simulink model "simuMF"  (R2021a)
settings: Solver=VariableStepAuto  StartTime=0.0  StopTime=100000  RelTol=1e-3
values from neighbouring files (symbols this model uses):
  C1 = tf(C1)    [control.m]
  C2 = tf(C2)    [control.m]
  H = tf(0.0001867, [1 0.0001919])    [control.m]
  pi_cd = tf(pi)    [control.m]
  pif = tf([39.15 0.06366], [1 0])    [control.m]
libraries: simulink x1
settings Model: Creator=jricl  LastModifiedBy=jricl

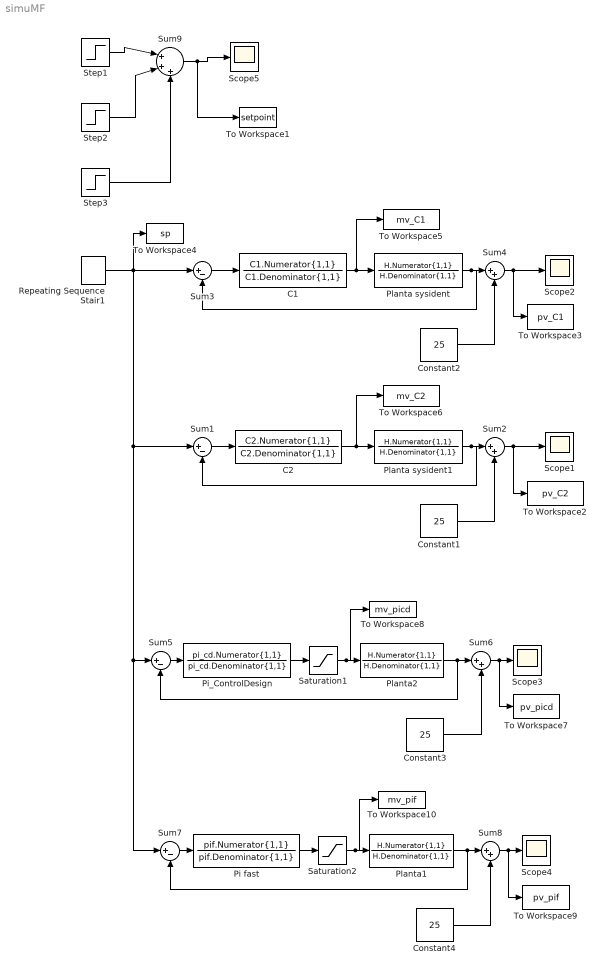
== system simuMF ==
  C1 : TransferFcn  Numerator=C1.Numerator{1,1}  Denominator=C1.Denominator{1,1}
  C2 : TransferFcn  Numerator=C2.Numerator{1,1}  Denominator=C2.Denominator{1,1}
  Constant{1..4} (4 alike) : Constant  Value=25
  Pi fast : TransferFcn  Numerator=pif.Numerator{1,1}  Denominator=pif.Denominator{1,1}
  Pi_ControlDesign : TransferFcn  Numerator=pi_cd.Numerator{1,1}  Denominator=pi_cd.Denominator{1,1}
  Planta sysident : TransferFcn  Numerator=H.Numerator{1,1}  Denominator=H.Denominator{1,1}
  Planta sysident1 : TransferFcn  Numerator=H.Numerator{1,1}  Denominator=H.Denominator{1,1}
  Planta1 : TransferFcn  Numerator=H.Numerator{1,1}  Denominator=H.Denominator{1,1}
  Planta2 : TransferFcn  Numerator=H.Numerator{1,1}  Denominator=H.Denominator{1,1}
  Repeating Sequence Stair1 : simulink/Sources/Repeating Sequence Stair  OutValues=[5 10 15 20]  tsamp=25000  OutMin=[]  OutMax=[]  OutDataTypeStr=double  OutputDataTypeScalingMode=double  OutDataType=fixdt(0,8)  ConRadixGroup=Best Precision: Vector-wise  OutScaling=2^-12
  Saturation1 : Saturate  UpperLimit=100  LowerLimit=0
  Saturation2 : Saturate  UpperLimit=100  LowerLimit=0
  Scope{1..5} (5 alike) : Scope
  Step1 : Step  Time=25000  Before=30  After=35
  Step2 : Step  Time=25000+25000  After=5
  Step3 : Step  Time=25000+25000+25000  After=5
  Sum{1,3,5,7} (4 alike) : Sum  Inputs=|+-
  Sum{2,4,6,8} (4 alike) : Sum  Inputs=|++
  Sum9 : Sum  Inputs=|+++
  To Workspace1 : ToWorkspace  VariableName=setpoint  SaveFormat=Timeseries  SampleTime=-1
  To Workspace10 : ToWorkspace  VariableName=mv_pif  SaveFormat=Timeseries  SampleTime=-1
  To Workspace2 : ToWorkspace  VariableName=pv_C2  SaveFormat=Timeseries  SampleTime=-1
  To Workspace3 : ToWorkspace  VariableName=pv_C1  SaveFormat=Timeseries  SampleTime=-1
  To Workspace4 : ToWorkspace  VariableName=sp  SaveFormat=Timeseries  SampleTime=-1
  To Workspace5 : ToWorkspace  VariableName=mv_C1  SaveFormat=Timeseries  SampleTime=-1
  To Workspace6 : ToWorkspace  VariableName=mv_C2  SaveFormat=Timeseries  SampleTime=-1
  To Workspace7 : ToWorkspace  VariableName=pv_picd  SaveFormat=Timeseries  SampleTime=-1
  To Workspace8 : ToWorkspace  VariableName=mv_picd  SaveFormat=Timeseries  SampleTime=-1
  To Workspace9 : ToWorkspace  VariableName=pv_pif  SaveFormat=Timeseries  SampleTime=-1
  wires:
  Constant2/1 -> Sum4/2
  Sum4/1 -> Scope2/1, To Workspace3/1
  Sum3/1 -> C1/1
  C1/1 -> Planta sysident/1, To Workspace5/1
  Planta sysident/1 -> Sum4/1, Sum3/2
  Step3/1 -> Sum9/3
  Step1/1 -> Sum9/1
  Sum9/1 -> To Workspace1/1, Scope5/1
  Step2/1 -> Sum9/2
  Planta sysident1/1 -> Sum1/2, Sum2/1
  C2/1 -> To Workspace6/1, Planta sysident1/1
  Sum1/1 -> C2/1
  Sum2/1 -> To Workspace2/1, Scope1/1
  Constant1/1 -> Sum2/2
  Sum6/1 -> Scope3/1, To Workspace7/1
  Constant3/1 -> Sum6/2
  Planta2/1 -> Sum5/2, Sum6/1
  Saturation1/1 -> To Workspace8/1, Planta2/1
  Sum5/1 -> Pi_ControlDesign/1
  Pi_ControlDesign/1 -> Saturation1/1
  Repeating Sequence Stair1/1 -> Sum1/1, Sum7/1, Sum5/1, Sum3/1, To Workspace4/1
  Pi fast/1 -> Saturation2/1
  Sum7/1 -> Pi fast/1
  Saturation2/1 -> Planta1/1, To Workspace10/1
  Planta1/1 -> Sum8/1, Sum7/2
  Constant4/1 -> Sum8/2
  Sum8/1 -> To Workspace9/1, Scope4/1
